simulink model "exercise1"  (R2017a)
settings: Solver=VariableStepAuto  StartTime=0.0  StopTime=20  RelTol=1e-3
settings Model: Creator=viktor  LastModifiedBy=viktor

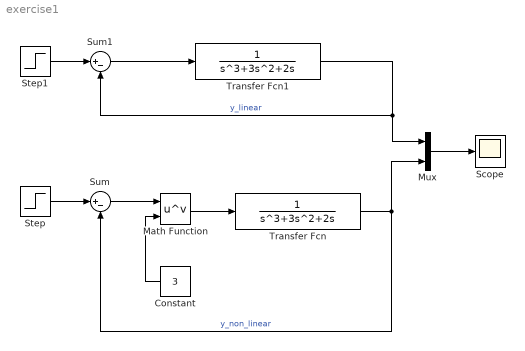
== system exercise1 ==
  Constant : Constant  Value=3
  Math Function : Math  Operator=pow  SaturateOnIntegerOverflow=on
  Mux : Mux  Inputs=2
  Scope : Scope
  Step : Step  SampleTime=0
  Step1 : Step  SampleTime=0
  Sum : Sum  Inputs=|+-
  Sum1 : Sum  Inputs=|+-
  Transfer Fcn : TransferFcn  Denominator=[1 3 2 0]
  Transfer Fcn1 : TransferFcn  Denominator=[1 3 2 0]
  wires:
  Step/1 -> Sum/1
  Sum/1 -> Math Function/1
  Transfer Fcn/1 -> Sum/2, Mux/2  "y_non_linear"
  Constant/1 -> Math Function/2
  Math Function/1 -> Transfer Fcn/1
  Step1/1 -> Sum1/1
  Transfer Fcn1/1 -> Mux/1, Sum1/2  "y_linear"
  Sum1/1 -> Transfer Fcn1/1
  Mux/1 -> Scope/1
